simulink model "BandPass_Sim"  (R2022b)
settings: Solver=VariableStepAuto  StartTime=0.0  StopTime=10  RelTol=1e-3
values from neighbouring files (symbols this model uses):
  amplitude_input = 1    [BP_config.m]
  denGs = [1 (10*wc_H+10*wc_L)/10 (10*wc_H*wc_L)/10]    [BP_config.m]
  denGz = cell2mat(Gz.Denominator)    [BP_config.m]
  numGs = [wc_L (wc_H*wc_L)/10]    [BP_config.m]
  numGz = numGz(2:end)    [BP_config.m]
  offset_input = 0    [BP_config.m]
  Ts = 1/f_sample    (= 0.000769230769231)    [BP_config.m]
  Tsim = 0.001*Ts    (= 7.69230769231e-07)    [BP_config.m]
  w_input = 2*pi*f_input    (= 62831.8530718)    [BP_config.m]
settings Model: Creator=mluser  LastModifiedBy=mluser
settings SFSimCC: SimCustomHeaderCode="#include \"BandPass.h\""  SimUserSources=BandPass.c  SimUserIncludeDirs=MATLAB Drive/Regulacion/Filtros/BandPass
settings RTWCC: RTWUseSimCustomCode=on  CustomHeaderCode="#include \"BandPass.h\""  CustomInclude=MATLAB Drive/Regulacion/Filtros/BandPass  CustomSource=BandPass.c

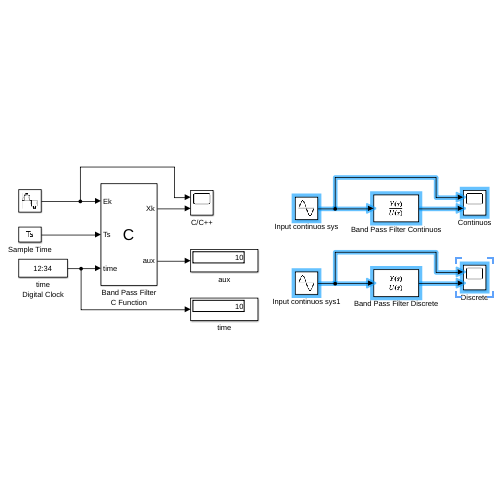
[thumbnail: Simulink's stored preview of the top-level diagram]
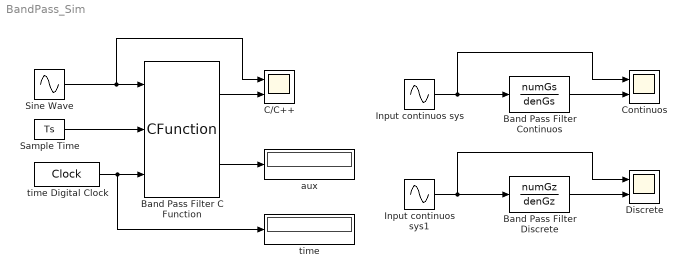
== system BandPass_Sim ==
  Band Pass Filter C Function : CFunction  OutputCode=Xk=BandPass(Ek, Ts, time, &aux);
  Band Pass Filter Continuos : TransferFcn  Description=Band Pass Filter  Numerator=numGs  Denominator=denGs
  Band Pass Filter Discrete : TransferFcn  Description=Band Pass Filter  Numerator=numGz  Denominator=denGz
  C/C++ : Scope  NumInputPorts=2
  Continuos : Scope  NumInputPorts=2
  Discrete : Scope  NumInputPorts=2
  Input continuos sys : Sin  Amplitude=amplitude_input  Bias=offset_input  Frequency=w_input  SampleTime=0
  Input continuos sys1 : Sin  Amplitude=amplitude_input  Bias=offset_input  Frequency=w_input  SampleTime=0
  Sample Time : Constant  Value=Ts
  Sine Wave : Sin  Amplitude=amplitude_input  Bias=offset_input  Frequency=w_input  SampleTime=Tsim
  aux : Display
  time : Display
  time Digital Clock : DigitalClock  SampleTime=Tsim
  wires:
  Input continuos sys/1 -> Continuos/1, Band Pass Filter Continuos/1
  Band Pass Filter Continuos/1 -> Continuos/2
  Sine Wave/1 -> C/C++/1, Band Pass Filter C Function/1
  Sample Time/1 -> Band Pass Filter C Function/2
  time Digital Clock/1 -> time/1, Band Pass Filter C Function/3
  Band Pass Filter C Function/1 -> C/C++/2
  Band Pass Filter C Function/2 -> aux/1
  Band Pass Filter Discrete/1 -> Discrete/2
  Input continuos sys1/1 -> Discrete/1, Band Pass Filter Discrete/1
